simulink model "gm_simpleController"  (R2020b)
settings: Solver=FixedStepDiscrete  StartTime=0.0  StopTime=10.0  RelTol=1e-3
libraries: hdlmdlgenlib x8
settings Model: Creator=amira  LastModifiedBy=amira
settings OptimizationCC: BlockReduction=off  ConditionallyExecuteInputs=off
settings DebuggingCC: InheritedTsInSrcMsg=none

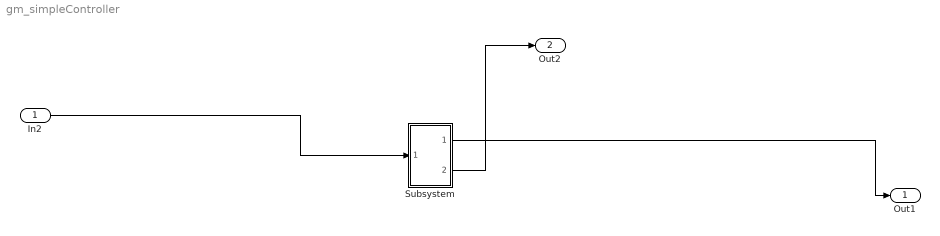
== system gm_simpleController ==
  In2 : Inport
  Subsystem : Subsystem
  Out1 : Outport  SignalName=C  VectorParamsAs1DForOutWhenUnconnected=off
  Out2 : Outport  Port=2  SignalName=U  VectorParamsAs1DForOutWhenUnconnected=off
  wires:
  Subsystem/2(Out2) -> Out2/1
  Subsystem/1(Out1) -> Out1/1
  In2/1 -> Subsystem/1(In2)

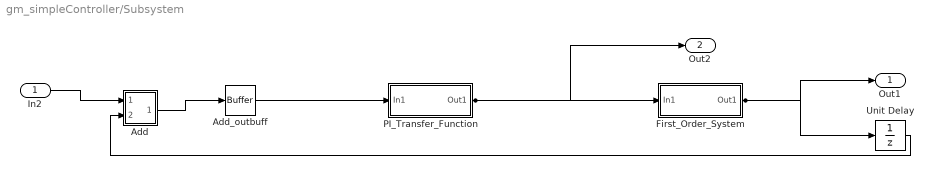
== system gm_simpleController/Subsystem ==
  In2 : Inport  OutDataTypeStr=single  PortDimensions=1  SampleTime=0.2
  Add : Subsystem
      mask Display: disp('NFP\nadd');
  Add_outbuff : hdlmdlgenlib/Buffer
      settings: SourceProductBaseCode=SL
  First_Order_System : Subsystem
  PI_Transfer_Function : Subsystem
  Unit Delay : UnitDelay  InitialCondition=single(0)  SampleTime=0.2
  Out1 : Outport  OutDataTypeStr=single  VectorParamsAs1DForOutWhenUnconnected=off
  Out2 : Outport  Port=2  OutDataTypeStr=single  VectorParamsAs1DForOutWhenUnconnected=off
  wires:
  In2/1 -> Add/1(In1)
  Add_outbuff/1 -> PI_Transfer_Function/1(In1)
  First_Order_System/1(Out1) -> Unit Delay/1, Out1/1
  PI_Transfer_Function/1(Out1) -> Out2/1, First_Order_System/1(In1)
  Unit Delay/1 -> Add/2(In2)
  Add/1(Out1) -> Add_outbuff/1

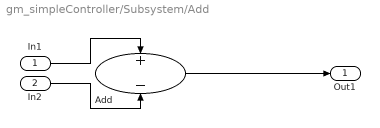
== system gm_simpleController/Subsystem/Add ==
  In1 : Inport
  In2 : Inport  Port=2
  Add : Sum  Inputs=+-  OutDataTypeStr=single  SampleTime=0.2
  Out1 : Outport
  wires:
  In1/1 -> Add/1
  In2/1 -> Add/2
  Add/1 -> Out1/1

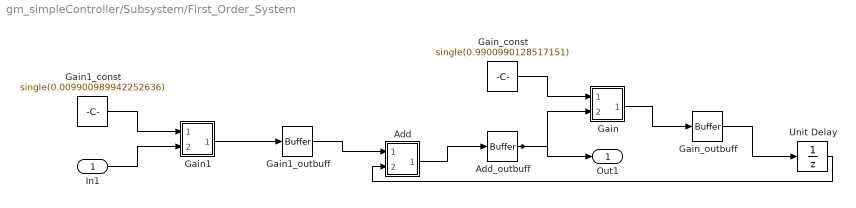
== system gm_simpleController/Subsystem/First_Order_System ==
  In1 : Inport  OutDataTypeStr=single  PortDimensions=1  SampleTime=0.2
  Add : Subsystem
      mask Display: disp('NFP\nadd');
  Add_outbuff : hdlmdlgenlib/Buffer
      settings: SourceProductBaseCode=SL
  Gain : Subsystem
      mask Display: disp('NFP\nmul');
  Gain1 : Subsystem
      mask Display: disp('NFP\nmul');
  Gain1_const : Constant  Value=single(0.009900989942252636)  OutDataTypeStr=single  SampleTime=0.2
  Gain1_outbuff : hdlmdlgenlib/Buffer
      settings: SourceProductBaseCode=SL
  Gain_const : Constant  Value=single(0.9900990128517151)  OutDataTypeStr=single  SampleTime=0.2
  Gain_outbuff : hdlmdlgenlib/Buffer
      settings: SourceProductBaseCode=SL
  Unit Delay : UnitDelay  InitialCondition=single(0)  SampleTime=0.2
  Out1 : Outport  VectorParamsAs1DForOutWhenUnconnected=off
  wires:
  In1/1 -> Gain1/2(In2)
  Add_outbuff/1 -> Gain/2(In2), Out1/1
  Gain_outbuff/1 -> Unit Delay/1
  Gain1_outbuff/1 -> Add/1(In1)
  Unit Delay/1 -> Add/2(In2)
  Gain_const/1 -> Gain/1(In1)
  Gain1_const/1 -> Gain1/1(In1)
  Add/1(Out1) -> Add_outbuff/1
  Gain/1(Out1) -> Gain_outbuff/1
  Gain1/1(Out1) -> Gain1_outbuff/1

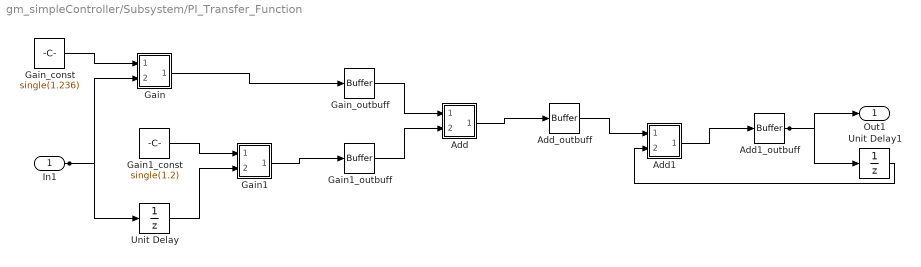
== system gm_simpleController/Subsystem/PI_Transfer_Function ==
  In1 : Inport  OutDataTypeStr=single  PortDimensions=1  SampleTime=0.2
  Add : Subsystem
      mask Display: disp('NFP\nadd');
  Add1 : Subsystem
      mask Display: disp('NFP\nadd');
  Add1_outbuff : hdlmdlgenlib/Buffer
      settings: SourceProductBaseCode=SL
  Add_outbuff : hdlmdlgenlib/Buffer
      settings: SourceProductBaseCode=SL
  Gain : Subsystem
      mask Display: disp('NFP\nmul');
  Gain1 : Subsystem
      mask Display: disp('NFP\nmul');
  Gain1_const : Constant  Value=single(1.2)  OutDataTypeStr=single  SampleTime=0.2
  Gain1_outbuff : hdlmdlgenlib/Buffer
      settings: SourceProductBaseCode=SL
  Gain_const : Constant  Value=single(1.236)  OutDataTypeStr=single  SampleTime=0.2
  Gain_outbuff : hdlmdlgenlib/Buffer
      settings: SourceProductBaseCode=SL
  Unit Delay : UnitDelay  InitialCondition=single(0)  SampleTime=0.2
  Unit Delay1 : UnitDelay  InitialCondition=single(0)  SampleTime=0.2
  Out1 : Outport  VectorParamsAs1DForOutWhenUnconnected=off
  wires:
  In1/1 -> Gain/2(In2), Unit Delay/1
  Add_outbuff/1 -> Add1/1(In1)
  Add1_outbuff/1 -> Unit Delay1/1, Out1/1
  Gain_outbuff/1 -> Add/1(In1)
  Gain1_outbuff/1 -> Add/2(In2)
  Unit Delay/1 -> Gain1/2(In2)
  Unit Delay1/1 -> Add1/2(In2)
  Gain_const/1 -> Gain/1(In1)
  Gain1_const/1 -> Gain1/1(In1)
  Add/1(Out1) -> Add_outbuff/1
  Add1/1(Out1) -> Add1_outbuff/1
  Gain/1(Out1) -> Gain_outbuff/1
  Gain1/1(Out1) -> Gain1_outbuff/1

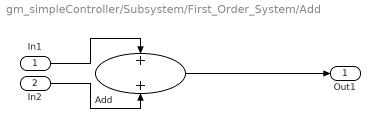
== system gm_simpleController/Subsystem/First_Order_System/Add ==
  In1 : Inport
  In2 : Inport  Port=2
  Add : Sum  OutDataTypeStr=single  SampleTime=0.2
  Out1 : Outport
  wires:
  In1/1 -> Add/1
  In2/1 -> Add/2
  Add/1 -> Out1/1

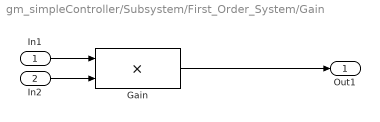
== system gm_simpleController/Subsystem/First_Order_System/Gain ==
  In1 : Inport
  In2 : Inport  Port=2
  Gain : Product  Inputs=**  OutDataTypeStr=single  SampleTime=0.2
  Out1 : Outport
  wires:
  In1/1 -> Gain/1
  In2/1 -> Gain/2
  Gain/1 -> Out1/1

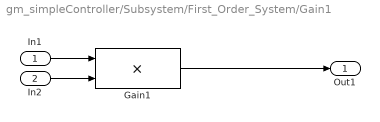
== system gm_simpleController/Subsystem/First_Order_System/Gain1 ==
  In1 : Inport
  In2 : Inport  Port=2
  Gain1 : Product  Inputs=**  OutDataTypeStr=single  SampleTime=0.2
  Out1 : Outport
  wires:
  In1/1 -> Gain1/1
  In2/1 -> Gain1/2
  Gain1/1 -> Out1/1

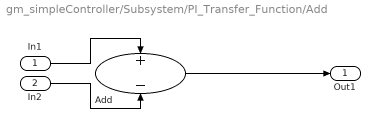
== system gm_simpleController/Subsystem/PI_Transfer_Function/Add ==
  In1 : Inport
  In2 : Inport  Port=2
  Add : Sum  Inputs=+-  OutDataTypeStr=single  SampleTime=0.2
  Out1 : Outport
  wires:
  In1/1 -> Add/1
  In2/1 -> Add/2
  Add/1 -> Out1/1

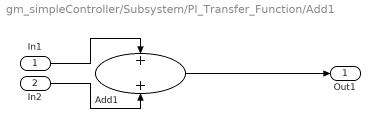
== system gm_simpleController/Subsystem/PI_Transfer_Function/Add1 ==
  In1 : Inport
  In2 : Inport  Port=2
  Add1 : Sum  OutDataTypeStr=single  SampleTime=0.2
  Out1 : Outport
  wires:
  In1/1 -> Add1/1
  In2/1 -> Add1/2
  Add1/1 -> Out1/1

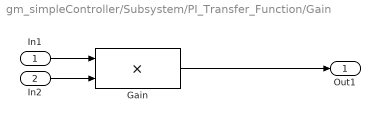
== system gm_simpleController/Subsystem/PI_Transfer_Function/Gain ==
  In1 : Inport
  In2 : Inport  Port=2
  Gain : Product  Inputs=**  OutDataTypeStr=single  SampleTime=0.2
  Out1 : Outport
  wires:
  In1/1 -> Gain/1
  In2/1 -> Gain/2
  Gain/1 -> Out1/1

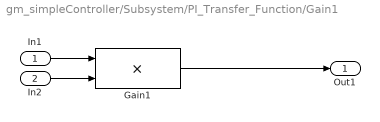
== system gm_simpleController/Subsystem/PI_Transfer_Function/Gain1 ==
  In1 : Inport
  In2 : Inport  Port=2
  Gain1 : Product  Inputs=**  OutDataTypeStr=single  SampleTime=0.2
  Out1 : Outport
  wires:
  In1/1 -> Gain1/1
  In2/1 -> Gain1/2
  Gain1/1 -> Out1/1
